simulink model "FIRfilter"  (R2021a)
settings: Solver=FixedStepAuto  StartTime=0.0  StopTime=20  RelTol=1e-3
settings Model: Creator=Asus  LastModifiedBy=Asus

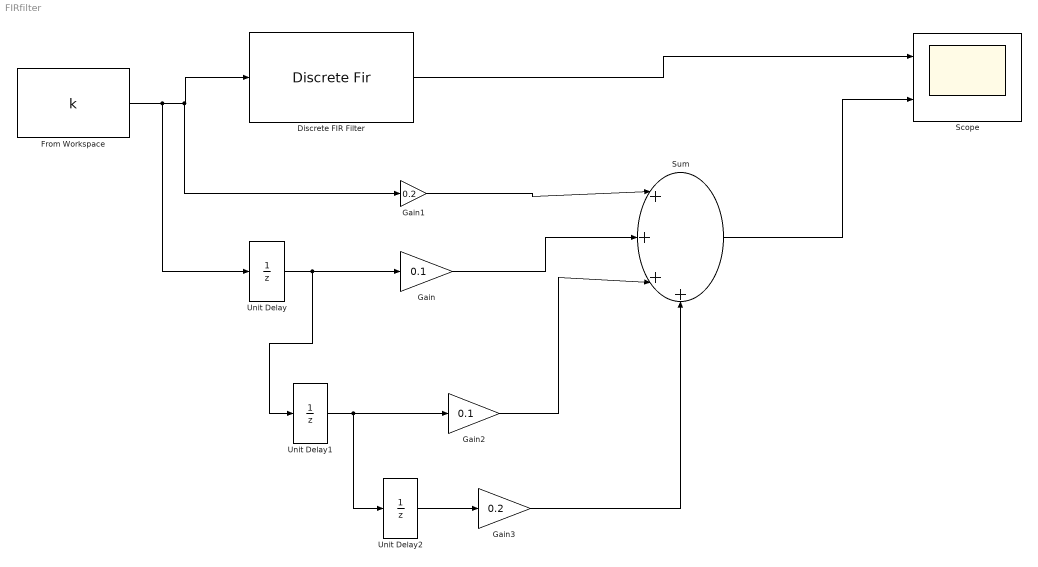
== system FIRfilter ==
  Discrete FIR Filter : DiscreteFir  Coefficients=[0.2 0.1 0.1 0.2 ]
  From Workspace : FromWorkspace  VariableName=k  SampleTime=-1
  Gain : Gain  Gain=0.1
  Gain1 : Gain  Gain=0.2
  Gain2 : Gain  Gain=0.1
  Gain3 : Gain  Gain=0.2
  Scope : Scope  NumInputPorts=2
  Sum : Sum  Inputs=|++++
  Unit Delay : UnitDelay  SampleTime=-1  HasFrameUpgradeWarning=on
  Unit Delay1 : UnitDelay  SampleTime=-1  HasFrameUpgradeWarning=on
  Unit Delay2 : UnitDelay  SampleTime=-1  HasFrameUpgradeWarning=on
  wires:
  From Workspace/1 -> Unit Delay/1, Gain1/1, Discrete FIR Filter/1
  Discrete FIR Filter/1 -> Scope/1
  Gain1/1 -> Sum/1
  Unit Delay/1 -> Unit Delay1/1, Gain/1
  Gain/1 -> Sum/2
  Unit Delay1/1 -> Unit Delay2/1, Gain2/1
  Gain2/1 -> Sum/3
  Unit Delay2/1 -> Gain3/1
  Gain3/1 -> Sum/4
  Sum/1 -> Scope/2
